simulink model "KUKA_EE_Trajectory_follower"  (R2021b)
settings: Solver=ode4  StartTime=0.0  StopTime=100  FixedStep=0.01  RelTol=1e-3
InitFcn:
  | %rho_0t=[0.29;0.29;0.29]; %m
  | %V_0t=[-0.001;-0.001;0];%[-0.0005;-0.0005;0];
  | %w_t=[0;0;-0.002];
  | 
  | 
  | %rho_0t=[0.3;0.3;0.2]; %m
  | %V_0t=[-0.001;-0.001;0];%[-0.0005;-0.0005;0];
  | %w_t=[0;0;-0.001];
values from neighbouring files (symbols this model uses):
  I0 = eye(3)*416.667    [Main.m]
  iota0 = eye(6,6)    [Internal_KUKA_Main.m]    (also in KUKA_Main.m; Main.m = [1 0 0; 0 1 0;zeros(3,3);0 0 1])
  K_d = 10*[1.3*eye(3) zeros(3);zeros(3) 0.8*eye(3)]    [Initiate_FQ.m]    (also in Internal_KUKA_Main.m = 200*[0.7*eye(3) zeros(3);zeros(3) 0.5*eye(3)]; KUKA_Main.m = [0.7*eye(3) zeros(3);zeros(3) 0.5*eye(3)])
  K_i = 5*[0.1*eye(3) zeros(3);zeros(3) 0.01*eye(3)]    [Initiate_FQ.m]    (also in Internal_KUKA_Main.m = 200*[0.01*eye(3) zeros(3);zeros(3) 0.001*eye(3)]; KUKA_Main.m = [0.01*eye(3) zeros(3);zeros(3) 0.001*eye(3)])
  K_p = 50*[0.1 0 0 0 0 0;0 0.1 0 0 0 0; 0 0 0.1 0 0 0; 0 0 0 0.01 0 0 ... (first row only)    [Initiate_FQ.m]    (also in Internal_KUKA_Main.m = 200*[0.1 0 0 0 0 0;0 0.1 0 0 0 0; 0 0 0.1 0 0 0; 0 0 0 0.01 ; KUKA_Main.m = [0.1 0 0 0 0 0;0 0.1 0 0 0 0; 0 0 0.1 0 0 0; 0 0 0 0.01 0 0)
  K_w = 20*eye(7)    [Initiate_FQ.m]
  K_wd = 1*eye(7)    [Initiate_FQ.m]
  M0 = M_temp.M0.data(:,:,1)    [Initiate_FQ.m]    (also in Internal_KUKA_Main.m; KUKA_Main.m)
  m0 = robot.Bodies{1,n+1}.Mass    [Internal_KUKA_Main.m]    (also in KUKA_Main.m; Main.m = 100)
  M0m = M_temp.M0m.data(:,:,1)    [Initiate_FQ.m]    (also in Internal_KUKA_Main.m; KUKA_Main.m)
  M_t = [eye(3)*mt zeros(3); zeros(3) eye(3)*0.416667]    [Initiate_FQ.m]    (also in Internal_KUKA_Main.m = [eye(3)*mt zeros(3); zeros(3) eye(3)*80]; KUKA_Main.m = [eye(3)*mt zeros(3); zeros(3) eye(3)*80])
  Mm = simplify(transpose(Xi_m)*transpose(Lm)*diagM*Lm*Xi_m)    [Internal_KUKA_Main.m]    (also in KUKA_Main.m)
  mm = zeros(1,n)    [Internal_KUKA_Main.m]    (also in KUKA_Main.m; Main.m = [2 2])
  mu = -10.*P0    [Initiate_FQ.m]    (also in Internal_KUKA_Main.m = P; KUKA_Main.m = P; Main.m = zeros(6,1)')
  mu_t = -10.*M_t*[V_0t;w_t]    [Initiate_FQ.m]    (also in Internal_KUKA_Main.m = M_t*[V_0t;w_t]; KUKA_Main.m = M_t*[V_0t;w_t])
  q_dot_m = 0.01*q_dot_m    [Initiate_FQ.m]    (also in Internal_KUKA_Main.m = [qdot1;qdot2;qdot3;qdot4;qdot5;qdot6;qdot7]; KUKA_Main.m = [qdot1;qdot2;qdot3;qdot4;qdot5;qdot6;qdot7]; Main.m = [0;0]; sendJointTorques.m = fread(t, 7, 'double'))
  q_m = [0.2;1.2;0.3;1.8;0.5;1.3;0.6]    [Initiate_FQ.m]    (also in Internal_KUKA_Main.m = [q_m1;q_m2;q_m3;q_m4;q_m5;q_m6;q_m7]; KUKA_Main.m = [q_m1;q_m2;q_m3;q_m4;q_m5;q_m6;q_m7]; Main.m = [0;0]; sendJointTorques.m = fread(t, 7, 'double'))
  rho_0t = [0;0;0.2]    [Initiate_FQ.m]    (also in Internal_KUKA_Main.m = [0.24;0.26;0.25]; KUKA_Main.m = [0.23;0.27;0.26])
  sc_size = 0    [Internal_KUKA_Main.m]    (also in KUKA_Main.m = 1)
  V_0t = -[-0.0005;-0.0005;0]    [Initiate_FQ.m]    (also in Internal_KUKA_Main.m = [-0.01;-0.01;0]; KUKA_Main.m = [-0.002;-0.002;0])
  V_I0 = 0.01*V_I0    [Initiate_FQ.m]    (also in Internal_KUKA_Main.m = [0;0;0;0;0;0]; KUKA_Main.m = [0;0;0;0;0;0]; Main.m = [0;0;0])
  X = [0 -x(3) x(2) ; x(3) 0 -x(1) ; -x(2) x(1) 0 ]    [skewsym.m]
  Xi_m = Xi_m(1:robot.n*6,1:robot.n)    [Internal_KUKA_Main.m]    (also in KUKA_Main.m)
  Xi_m_matrix = zeros(6*n,n)    [Internal_KUKA_Main.m]    (also in KUKA_Main.m; Main.m)
undefined symbols (not defined in the file or in its folder): fall_distance, g_cm, g_cm0, Ie, Im, m0_frak, m_diag, me, rise_time, Y, Z
libraries: nesl_utility x178, sm_lib x175, robotcorelib x7
(part 4 of 8)

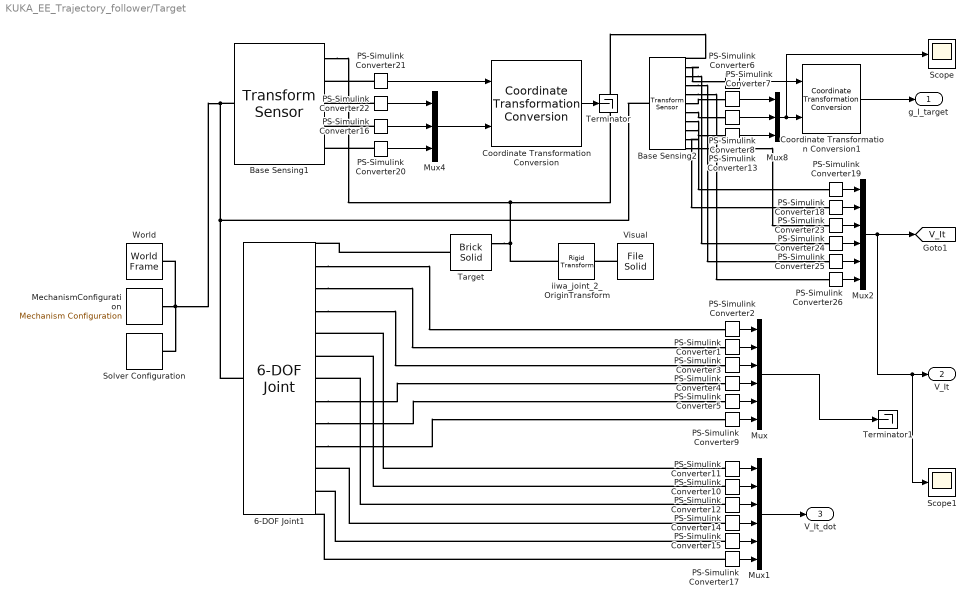
== system KUKA_EE_Trajectory_follower/Target ==
  6-DOF Joint1 : sm_lib/Joints/6-DOF Joint  JointMode=Normal  SenseConstraintForce=off  SenseConstraintForceX=off  SenseConstraintForceY=off  SenseConstraintForceZ=off  SenseConstraintTorque=off  SenseConstraintTorqueX=off  SenseConstraintTorqueY=off  SenseConstraintTorqueZ=off  SenseTotalForce=off  SenseTotalForceX=off  SenseTotalForceY=off  SenseTotalForceZ=off  SenseTotalTorque=off  SenseTotalTorqueX=off  SenseTotalTorqueY=off  SenseTotalTorqueZ=off  CompositeWrenchDir=FollowerOnBase  CompositeWrenchFrame=BaseFrame  PxEquilibriumPosition=0  PxEquilibriumPositionUnits=m  PxSpringStiffness=0  PxSpringStiffnessUnits=N/m  PxDampingCoefficient=0  PxDampingCoefficientUnits=N/(m/s)  PxTorqueActuationMode=NoTorque  PxMotionActuationMode=ComputedMotion  PxSensePosition=off  PxSenseVelocity=on  PxSenseAcceleration=on  PxSenseTorqueForce=off  PxSenseLowerLimitTorqueForce=off  PxSenseUpperLimitTorqueForce=off  PxLowerLimitSpecify=off  PxLowerLimitBound=-1  PxLowerLimitBoundUnits=m  PxLowerLimitStiffness=1e6  PxLowerLimitStiffnessUnits=N/m  PxLowerLimitDamping=1e3  PxLowerLimitDampingUnits=N/(m/s)  PxLowerLimitTransitionRegionWidth=1e-4  PxLowerLimitTransitionRegionWidthUnits=m  PxUpperLimitSpecify=off  PxUpperLimitBound=1  PxUpperLimitBoundUnits=m  PxUpperLimitStiffness=1e6  PxUpperLimitStiffnessUnits=N/m  PxUpperLimitDamping=1e3  PxUpperLimitDampingUnits=N/(m/s)  PxUpperLimitTransitionRegionWidth=1e-4  PxUpperLimitTransitionRegionWidthUnits=m  PxPositionTargetSpecify=on  PxPositionTargetPriority=High  PxPositionTargetValue=rho_0t(1)  PxPositionTargetValueUnits=m  PxVelocityTargetSpecify=on  PxVelocityTargetPriority=High  PxVelocityTargetValue=V_0t(1)  PxVelocityTargetValueUnits=m/s  PyEquilibriumPosition=0  PyEquilibriumPositionUnits=m  PySpringStiffness=0  PySpringStiffnessUnits=N/m  PyDampingCoefficient=0  PyDampingCoefficientUnits=N/(m/s)  PyTorqueActuationMode=NoTorque  PyMotionActuationMode=ComputedMotion  PySensePosition=off  PySenseVelocity=on  PySenseAcceleration=on  PySenseTorqueForce=off  PySenseLowerLimitTorqueForce=off  PySenseUpperLimitTorqueForce=off  PyLowerLimitSpecify=off  PyLowerLimitBound=-1  PyLowerLimitBoundUnits=m  PyLowerLimitStiffness=1e6  PyLowerLimitStiffnessUnits=N/m  PyLowerLimitDamping=1e3  PyLowerLimitDampingUnits=N/(m/s)  PyLowerLimitTransitionRegionWidth=1e-4  PyLowerLimitTransitionRegionWidthUnits=m  PyUpperLimitSpecify=off  PyUpperLimitBound=1  PyUpperLimitBoundUnits=m  PyUpperLimitStiffness=1e6  PyUpperLimitStiffnessUnits=N/m  PyUpperLimitDamping=1e3  PyUpperLimitDampingUnits=N/(m/s)  PyUpperLimitTransitionRegionWidth=1e-4  PyUpperLimitTransitionRegionWidthUnits=m  PyPositionTargetSpecify=on  PyPositionTargetPriority=High  PyPositionTargetValue=rho_0t(2)  PyPositionTargetValueUnits=m  PyVelocityTargetSpecify=on  PyVelocityTargetPriority=High  PyVelocityTargetValue=V_0t(2)  PyVelocityTargetValueUnits=m/s  PzEquilibriumPosition=0  PzEquilibriumPositionUnits=m  PzSpringStiffness=0  PzSpringStiffnessUnits=N/m  PzDampingCoefficient=0  PzDampingCoefficientUnits=N/(m/s)  PzTorqueActuationMode=NoTorque  PzMotionActuationMode=ComputedMotion  PzSensePosition=off  PzSenseVelocity=on  PzSenseAcceleration=on  PzSenseTorqueForce=off  PzSenseLowerLimitTorqueForce=off  PzSenseUpperLimitTorqueForce=off  PzLowerLimitSpecify=off  PzLowerLimitBound=-1  PzLowerLimitBoundUnits=m  PzLowerLimitStiffness=1e6  PzLowerLimitStiffnessUnits=N/m  PzLowerLimitDamping=1e3  PzLowerLimitDampingUnits=N/(m/s)  PzLowerLimitTransitionRegionWidth=1e-4  PzLowerLimitTransitionRegionWidthUnits=m  PzUpperLimitSpecify=off  PzUpperLimitBound=1  PzUpperLimitBoundUnits=m  PzUpperLimitStiffness=1e6  PzUpperLimitStiffnessUnits=N/m  PzUpperLimitDamping=1e3  PzUpperLimitDampingUnits=N/(m/s)  PzUpperLimitTransitionRegionWidth=1e-4  PzUpperLimitTransitionRegionWidthUnits=m  PzPositionTargetSpecify=on  PzPositionTargetPriority=High  PzPositionTargetValue=rho_0t(3)  PzPositionTargetValueUnits=m  PzVelocityTargetSpecify=on  PzVelocityTargetPriority=High  PzVelocityTargetValue=V_0t(3)  PzVelocityTargetValueUnits=m/s  SphDefPosRotationMethod=None  SphDefPosRotationAngleUnits=deg  SphDefPosRotationStandardAxis=+Z  SphDefPosRotationAngle=0.0  SphDefPosRotationArbitraryAxis=[0 0 1]  SphDefPosFollAlignAxisA=+X  SphDefPosBaseAlignAxisA=+Y  SphDefPosFollAlignAxisB=+Y  SphDefPosBaseAlignAxisB=+Z  SphDefPosRotationSequenceAxes=FollowerAxes  SphDefPosRotationSequence=XYX  SphDefPosRotationSequenceAngles=[0 0 0]  SphDefPosRotationSequenceAnglesUnits=deg  SphDefPosRotationMatrix=[1 0 0; 0 1 0; 0 0 1]  SphEqPosRotationMethod=None  SphEqPosRotationAngleUnits=deg  SphEqPosRotationStandardAxis=+Z  SphEqPosRotationAngle=0.0  SphEqPosRotationArbitraryAxis=[0 0 1]  SphEqPosFollAlignAxisA=+X  SphEqPosBaseAlignAxisA=+Y  SphEqPosFollAlignAxisB=+Y  SphEqPosBaseAlignAxisB=+Z  SphEqPosRotationSequenceAxes=FollowerAxes  SphEqPosRotationSequence=XYX  SphEqPosRotationSequenceAngles=[0 0 0]  SphEqPosRotationSequenceAnglesUnits=deg  SphEqPosRotationMatrix=[1 0 0; 0 1 0; 0 0 1]  SphSpringStiffness=0  SphSpringStiffnessUnits=N*m/deg  SphDampingCoefficient=0  SphDampingCoefficientUnits=N*m/(deg/s)  SphActuateTorqueX=off  SphActuateTorqueY=off  SphActuateTorqueZ=off  SphActuateTorque=off  SphTorqueActuationMode=NoTorque  SphMotionActuationMode=ComputedMotion  SphActuationFrame=BaseFrame  SphSensePosition=off  SphSenseVelocityX=on  SphSenseVelocityY=on  SphSenseVelocityZ=on  SphSenseVelocity=off  SphSenseAccelerationX=on  SphSenseAccelerationY=on  SphSenseAccelerationZ=on  SphSenseAcceleration=off  SphSenseTorqueX=off  SphSenseTorqueY=off  SphSenseTorqueZ=off  SphSenseTorqueForce=off  SphSenseLowerLimitTorqueMag=off  SphSenseUpperLimitTorqueMag=off  SphSensingFrame=BaseFrame  SphLowerLimitSpecify=off  SphLowerLimitBound=15  SphLowerLimitBoundUnits=deg  SphLowerLimitStiffness=1e4  SphLowerLimitStiffnessUnits=N*m/deg  SphLowerLimitDamping=10  SphLowerLimitDampingUnits=N*m/(deg/s)  SphLowerLimitTransitionRegionWidth=0.1  SphLowerLimitTransitionRegionWidthUnits=deg  SphUpperLimitSpecify=off  SphUpperLimitBound=45  SphUpperLimitBoundUnits=deg  SphUpperLimitStiffness=1e4  SphUpperLimitStiffnessUnits=N*m/deg  SphUpperLimitDamping=10  SphUpperLimitDampingUnits=N*m/(deg/s)  SphUpperLimitTransitionRegionWidth=0.1  SphUpperLimitTransitionRegionWidthUnits=deg  SphPositionTargetRotationMethod=RotationSequence  SphPositionTargetRotationAngleUnits=deg  SphPositionTargetRotationStandardAxis=+Z  SphPositionTargetRotationAngle=0.0  SphPositionTargetRotationArbitraryAxis=[0 0 1]  SphPositionTargetFollAlignAxisA=+X  SphPositionTargetBaseAlignAxisA=+Y  SphPositionTargetFollAlignAxisB=+Y  SphPositionTargetBaseAlignAxisB=+Z  SphPositionTargetRotationSequenceAxes=FollowerAxes  SphPositionTargetRotationSequence=XYZ  SphPositionTargetRotationSequenceAngles=[0 0 0]  SphPositionTargetRotationSequenceAnglesUnits=deg  SphPositionTargetRotationMatrix=[1 0 0; 0 1 0; 0 0 1]  SphPositionTargetSpecify=on  SphPositionTargetPriority=High  SphVelocityTargetValue=w_t  SphVelocityTargetValueUnits=rad/s  SphVelocityTargetSpecify=on  SphVelocityTargetPriority=High  SphVelocityTargetInFollowerFrame=off
  Base Sensing1 : sm_lib/Frames and Transforms/Transform Sensor  MeasurementFrame=Base  SenseAngle=off  SenseAxis=off  SenseAngle1=off  SenseAngle2=off  SenseAngle3=off  SenseQ=off  SenseR=on  SenseOmegaX=off  SenseOmegaY=off  SenseOmegaZ=off  SenseOmega1=off  SenseOmega2=off  SenseOmega3=off  SenseQDot=off  SenseRDot=off  SenseAlphaX=off  SenseAlphaY=off  SenseAlphaZ=off  SenseAlpha1=off  SenseAlpha2=off  SenseAlpha3=off  SenseQDDot=off  SenseRDDot=off  SenseX=on  SenseY=on  SenseZ=on  SenseRad=off  SenseAzim=off  SenseDist=off  SenseInc=off  SenseXDot=off  SenseYDot=off  SenseZDot=off  SenseRadDot=off  SenseAzimDot=off  SenseDistDot=off  SenseIncDot=off  SenseXDDot=off  SenseYDDot=off  SenseZDDot=off  SenseRadDDot=off  SenseAzimDDot=off  SenseDistDDot=off  SenseIncDDot=off
  Base Sensing2 : sm_lib/Frames and Transforms/Transform Sensor  MeasurementFrame=Base  SenseAngle=off  SenseAxis=off  SenseAngle1=off  SenseAngle2=off  SenseAngle3=off  SenseQ=off  SenseR=on  SenseOmegaX=on  SenseOmegaY=on  SenseOmegaZ=on  SenseOmega1=off  SenseOmega2=off  SenseOmega3=off  SenseQDot=off  SenseRDot=off  SenseAlphaX=off  SenseAlphaY=off  SenseAlphaZ=off  SenseAlpha1=off  SenseAlpha2=off  SenseAlpha3=off  SenseQDDot=off  SenseRDDot=off  SenseX=on  SenseY=on  SenseZ=on  SenseRad=off  SenseAzim=off  SenseDist=off  SenseInc=off  SenseXDot=on  SenseYDot=on  SenseZDot=on  SenseRadDot=off  SenseAzimDot=off  SenseDistDot=off  SenseIncDot=off  SenseXDDot=off  SenseYDDot=off  SenseZDDot=off  SenseRadDDot=off  SenseAzimDDot=off  SenseDistDDot=off  SenseIncDDot=off
  Coordinate Transformation Conversion : robotcorelib/Coordinate Transformation Conversion  InputRepresentation=Rotation Matrix  InputEulerSequence=ZYX  ShowTrVecInputPort=on  OutputRepresentation=Homogeneous Transformation  OutputEulerSequence=ZYX  ShowTrVecOutputPort=on  SimulateUsing=Interpreted execution
      settings: SourceProductBaseCode=NV,RO,RR,UV
  Coordinate Transformation Conversion1 : robotcorelib/Coordinate Transformation Conversion  InputRepresentation=Rotation Matrix  InputEulerSequence=ZYX  ShowTrVecInputPort=on  OutputRepresentation=Homogeneous Transformation  OutputEulerSequence=ZYX  ShowTrVecOutputPort=on  SimulateUsing=Interpreted execution
      settings: SourceProductBaseCode=NV,RO,RR,UV
  MechanismConfiguration : sm_lib/Utilities/Mechanism Configuration  UniformGravity=Constant  GravityVector=[0 0 0]  GravityUnits=m/s^2  LinearizationDelta=0.001  JointModeTransitionNonlinearIterations=2
  Mux : Mux  Inputs=6
  Mux1 : Mux  Inputs=6
  Mux2 : Mux  Inputs=6
  Mux4 : Mux  Inputs=3
  Mux8 : Mux  Inputs=3
  PS-Simulink Converter{1..26} (26 alike) : nesl_utility/PS-Simulink Converter  PhysicalDomain=network_engine_domain  SubClassName=ps_output  LeftPortType=input  RightPortType=output  PseudoPeriodic=off  Frequencies=[]  Unit=inherit  AffineConversion=off
      settings: SourceProductBaseCode=PW,SS
  Scope : Scope
  Scope1 : Scope
  Solver Configuration : nesl_utility/Solver Configuration  PhysicalDomain=network_engine_domain  SubClassName=solver  LeftPortType=input  RightPortType=generic  Tones=[]  Harmonics=[]  SimulateNoise=off  Profile=off  UseLocalSampling=off  EnableSwitchedLinearOptims=on  FrequencyDomain=off  UseCCode=off  RelTol=0.001  AbsTol=0.001  MinStep=1e-09  ToWorkspace=off  RevertToSquareIcSolve=off  NumHomotopyIterations=100  PhasorMode=off  PhasorModeNumHarmonics=1  DoDC=off  ResidualTolerance=1e-09  UseLocalSolver=off  LocalSolverChoice=NE_BACKWARD_EULER_ADVANCER  LocalSolverSampleTime=0.001  DoFixedCost=off  MaxNonlinIter=3  MaxModeIter=2  ComputeImpulses=off  ImpulseIterations=2  LinearAlgebra=Full  EquationFormulation=NE_TIME_EF  DelaysMemoryBudget=1024  AutomaticFiltering=on  FilteringTimeConstant=0.001  PartitionStorageMethod=AS_NEEDED  PartitionMemoryBudget=1024  PartitionMethod=ROBUST
      settings: SourceProductBaseCode=PW,SS
  Target : sm_lib/Body Elements/Brick Solid  GraphicAmbientColor=[0.15 0.15 0.15 1.0]  BasedOnType=Mass  BrickDimensions=[0.5, 0.5, 0.5]  BrickDimensionUnits=m  CenterOfMass=[0 0 0]  CenterOfMassUnits=m  GraphicDiffuseColor=[0.5 0.5 0.5]  Density=1000  DensityUnits=kg/m^3  DoExposeReferenceFrame=on  GraphicEmissiveColor=[0.0 0.0 0.0 1.0]  ExportEntireGeometry=on  SerializedFrames=<Frames><Frame><Id>Frame1</Id><Value><Name>F1</Name><Origin><Source>GeometricFeature</Source><FeatureName>-x -y -z point</FeatureName></Origin><PrimaryAxis><DefinedDirection>+Z</DefinedDirection><Source>ReferenceFrame</Source><SourceDirection>+Z</SourceDirection><FeatureName></FeatureName></PrimaryAxis><SecondaryAxis><DefinedDirection>+X</DefinedDirection><Source>ReferenceFrame</Source><SourceDirection>+X</SourceDirection><FeatureName></FeatureName></SecondaryAxis></Value></Frame></Frames>  MarkerShape=Sphere  MarkerSize=10  GraphicType=None  InertiaType=CalculateFromGeometry  Mass=10  MassUnits=kg  MomentsOfInertia=[1 1 1]  MomentsOfInertiaUnits=kg*m^2  GraphicOpacity=1.0  ProductsOfInertia=[0 0 0]  ProductsOfInertiaUnits=kg*m^2  GraphicShininess=75  GraphicSpecularColor=[0.5 0.5 0.5 1.0]  GraphicVisPropType=SimpleVisualProperties
  Terminator : Terminator
  Terminator1 : Terminator
  Visual : sm_lib/Body Elements/File Solid  ExtGeomFileName=Spacecrafts/CubeSatAssembly.stl  UnitType=Custom  ExtGeomFileUnits=cm  StepReaderType=HEX  ExportConvexHullGeometry=off  InertiaType=Custom  Mass=0  MassUnits=kg  CenterOfMass=[0, 0, 0]  CenterOfMassUnits=m  MomentsOfInertia=[0, 0, 0]  MomentsOfInertiaUnits=kg*m^2  ProductsOfInertia=[0, 0, 0]  ProductsOfInertiaUnits=kg*m^2  BasedOnType=DensityFromFile  Density=1000  DensityUnits=kg/m^3  DoExposeReferenceFrame=on  SerializedFrames=<Frames/>  GraphicType=FromGeometry  MarkerShape=Sphere  MarkerSize=10  GraphicVisPropType=SimpleVisualProperties  GraphicDiffuseColor=[0.4 0.4 0.4]  GraphicSpecularColor=[0.5 0.5 0.5 1.0]  GraphicAmbientColor=[0.15 0.15 0.15 1.0]  GraphicEmissiveColor=[0.0 0.0 0.0 1.0]  GraphicShininess=75  GraphicOpacity=1
  World : sm_lib/Frames and Transforms/World Frame
  iiwa_joint_2_OriginTransform : sm_lib/Frames and Transforms/Rigid Transform  TranslationMethod=Cartesian  TranslationStandardOffset=0  TranslationLengthUnit=m  TranslationStandardAxis=+Z  TranslationCartesianOffset=[-3.28, -4.43, 0.817]  TranslationROffset=0  TranslationROffsetUnits=m  TranslationZOffset=0  TranslationZOffsetUnits=m  TranslationThetaOffset=0  TranslationThetaOffsetUnits=deg  RotationMethod=RotationSequence  RotationAngleUnits=deg  RotationStandardAxis=+Z  RotationAngle=0.0  RotationArbitraryAxis=[0 0 1]  FollAlignAxisA=+X  BaseAlignAxisA=+Y  FollAlignAxisB=+Y  BaseAlignAxisB=+Z  RotationSequenceAxes=FollowerAxes  RotationSequence=XYZ  RotationSequenceAngles=[0 0 0]  RotationSequenceAnglesUnits=rad  RotationMatrix=[1 0 0; 0 1 0; 0 0 1]
  g_I_target : Outport
  V_It : Outport  Port=2
  V_It_dot : Outport  Port=3
  tag scope: V_It=global
  wires:
  PS-Simulink Converter20/1 -> Mux4/3
  PS-Simulink Converter13/1 -> Mux8/3
  PS-Simulink Converter4/1 -> Mux/4
  PS-Simulink Converter9/1 -> Mux/6
  PS-Simulink Converter3/1 -> Mux/3
  Coordinate Transformation Conversion/1 -> Terminator/1
  Mux1/1 -> V_It_dot/1
  PS-Simulink Converter16/1 -> Mux4/2
  Coordinate Transformation Conversion1/1 -> g_I_target/1
  PS-Simulink Converter11/1 -> Mux1/1
  PS-Simulink Converter1/1 -> Mux/2
  PS-Simulink Converter15/1 -> Mux1/5
  PS-Simulink Converter14/1 -> Mux1/4
  PS-Simulink Converter2/1 -> Mux/1
  PS-Simulink Converter7/1 -> Mux8/1
  PS-Simulink Converter21/1 -> Coordinate Transformation Conversion/1
  PS-Simulink Converter10/1 -> Mux1/2
  PS-Simulink Converter6/1 -> Coordinate Transformation Conversion1/1
  PS-Simulink Converter17/1 -> Mux1/6
  Mux4/1 -> Coordinate Transformation Conversion/2
  PS-Simulink Converter12/1 -> Mux1/3
  PS-Simulink Converter5/1 -> Mux/5
  PS-Simulink Converter22/1 -> Mux4/1
  PS-Simulink Converter8/1 -> Mux8/2
  Mux8/1 -> Scope/1, Coordinate Transformation Conversion1/2
  PS-Simulink Converter24/1 -> Mux2/4
  PS-Simulink Converter18/1 -> Mux2/2
  PS-Simulink Converter25/1 -> Mux2/5
  Mux2/1 -> Scope1/1, V_It/1, [V_It]
  PS-Simulink Converter19/1 -> Mux2/1
  PS-Simulink Converter23/1 -> Mux2/3
  PS-Simulink Converter26/1 -> Mux2/6
  Mux/1 -> Terminator1/1
  connections:
  Target/RConn1 -- 6-DOF Joint1/RConn1
  Base Sensing2/RConn2 -- PS-Simulink Converter6/LConn1
  PS-Simulink Converter15/LConn1 -- 6-DOF Joint1/RConn12
  6-DOF Joint1/RConn10 -- PS-Simulink Converter9/LConn1
  PS-Simulink Converter10/LConn1 -- 6-DOF Joint1/RConn6
  PS-Simulink Converter22/LConn1 -- Base Sensing1/RConn3
  Base Sensing2/RConn3 -- PS-Simulink Converter24/LConn1
  PS-Simulink Converter20/LConn1 -- Base Sensing1/RConn5
  World/RConn1 -- Base Sensing2/LConn1 -- 6-DOF Joint1/LConn1 -- Base Sensing1/LConn1 -- MechanismConfiguration/RConn1 -- Solver Configuration/RConn1
  PS-Simulink Converter21/LConn1 -- Base Sensing1/RConn2
  PS-Simulink Converter16/LConn1 -- Base Sensing1/RConn4
  Base Sensing2/RConn5 -- PS-Simulink Converter26/LConn1
  PS-Simulink Converter12/LConn1 -- 6-DOF Joint1/RConn7
  6-DOF Joint1/RConn9 -- PS-Simulink Converter5/LConn1
  6-DOF Joint1/RConn2 -- PS-Simulink Converter2/LConn1
  PS-Simulink Converter17/LConn1 -- 6-DOF Joint1/RConn13
  6-DOF Joint1/RConn4 -- PS-Simulink Converter3/LConn1
  PS-Simulink Converter14/LConn1 -- 6-DOF Joint1/RConn11
  6-DOF Joint1/RConn8 -- PS-Simulink Converter4/LConn1
  PS-Simulink Converter11/LConn1 -- 6-DOF Joint1/RConn5
  6-DOF Joint1/RConn3 -- PS-Simulink Converter1/LConn1
  Visual/RConn1 -- iiwa_joint_2_OriginTransform/RConn1
  Base Sensing2/RConn4 -- PS-Simulink Converter25/LConn1
  Base Sensing2/RConn6 -- PS-Simulink Converter7/LConn1
  Base Sensing2/RConn7 -- PS-Simulink Converter8/LConn1
  Base Sensing2/RConn8 -- PS-Simulink Converter13/LConn1
  Base Sensing2/RConn9 -- PS-Simulink Converter19/LConn1
  Base Sensing2/RConn10 -- PS-Simulink Converter18/LConn1
  Base Sensing2/RConn11 -- PS-Simulink Converter23/LConn1
  iiwa_joint_2_OriginTransform/LConn1 -- Target/LConn1 -- Base Sensing1/RConn1 -- Base Sensing2/RConn1

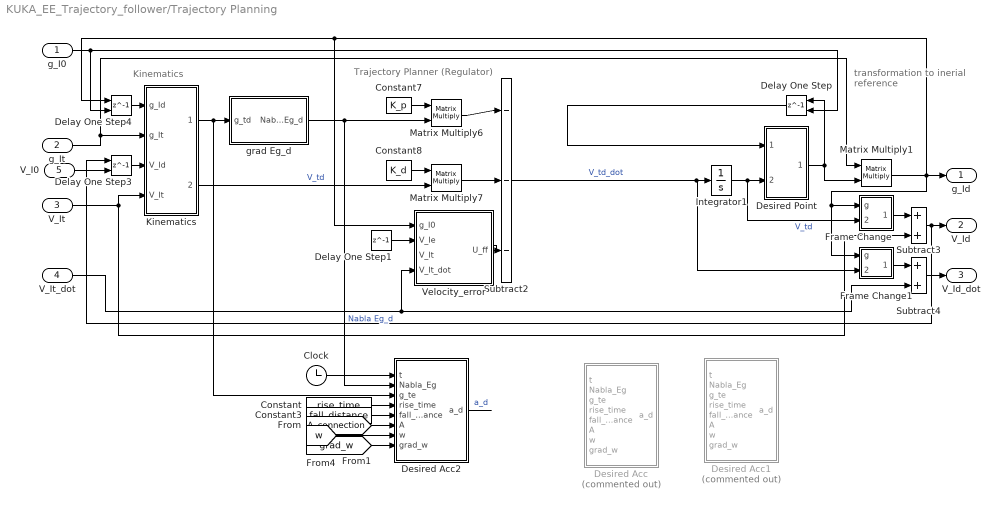
== system KUKA_EE_Trajectory_follower/Trajectory Planning ==
  note: Trajectory Planner (Regulator)
  note: Kinematics
  note: transformation
      | to inerial reference
  g_I0 : Inport
  g_It : Inport  Port=2
  V_It : Inport  Port=3
  V_It_dot : Inport  Port=4
  V_I0 : Inport  Port=5
  Clock : Clock
  Constant : Constant  Value=rise_time
  Constant3 : Constant  Value=fall_distance
  Constant7 : Constant  Value=K_p
  Constant8 : Constant  Value=K_d
  Delay One Step{,1,3..4} (4 alike) : Delay  DelayLength=1  InitialConditionSource=Input port
      settings: InputPortMap=u0,p4
  Desired Acc : MATLAB Function  Commented=on  TreatAsAtomicUnit=on
  Desired Acc1 : MATLAB Function  Commented=on  TreatAsAtomicUnit=on
  Desired Acc2 : MATLAB Function  TreatAsAtomicUnit=on
  Desired Point : MATLAB Function  TreatAsAtomicUnit=on
  Frame Change : MATLAB Function  TreatAsAtomicUnit=on
  Frame Change1 : MATLAB Function  TreatAsAtomicUnit=on
  Integrator1 : Integrator
  Kinematics : Subsystem
  Matrix Multiply1 : Product  Multiplication=Matrix(*)
  Matrix Multiply6 : Product  Multiplication=Matrix(*)
  Matrix Multiply7 : Product  Multiplication=Matrix(*)
  Subtract2 : Sum  Inputs=---
  Subtract3 : Sum
  Subtract4 : Sum
  Velocity_error : MATLAB Function  TreatAsAtomicUnit=on
  grad Eg_d : MATLAB Function  TreatAsAtomicUnit=on
  g_Id : Outport
  V_Id : Outport  Port=2
  V_Id_dot : Outport  Port=3
  wires:
  Constant3/1 -> Desired Acc2/5(fall_distance)
  Clock/1 -> Desired Acc2/1(t)
  [A_connection] -> Desired Acc2/6(A)
  [grad_w] -> Desired Acc2/8(grad_w)
  Constant/1 -> Desired Acc2/4(rise_time)
  Desired Acc2/1(a_d) -> ?  "a_d"
  [w] -> Desired Acc2/7(w)
  Kinematics/1(g_td) -> Desired Acc2/3(g_te), grad Eg_d/1(g_td)
  V_It/1 -> Subtract3/2, Kinematics/4(V_It)
  grad Eg_d/1(Nabla_Eg_d) -> Desired Acc2/2(Nabla_Eg), Matrix Multiply6/2  "Nabla Eg_d"
  g_It/1 -> Matrix Multiply1/1, Kinematics/2(g_It)
  Delay One Step3/1 -> Kinematics/3(V_Id)
  Kinematics/2(V_td) -> Matrix Multiply7/2  "V_td"
  Delay One Step/1 -> Desired Point/1(g_prev)
  V_I0/1 -> Delay One Step3/2
  Velocity_error/1(U_ff) -> Subtract2/3
  Constant8/1 -> Matrix Multiply7/1
  Matrix Multiply7/1 -> Subtract2/2
  Constant7/1 -> Matrix Multiply6/1
  V_It_dot/1 -> Velocity_error/4(V_It_dot), Subtract4/2
  Integrator1/1 -> Desired Point/2(V_d), Frame Change/2(A_in)  "V_td"
  g_I0/1 -> Delay One Step4/2, Delay One Step/2
  Matrix Multiply6/1 -> Subtract2/1
  Subtract2/1 -> Frame Change1/2(A_in), Integrator1/1  "V_td_dot"
  Desired Point/1(g_td) -> Matrix Multiply1/2, Delay One Step/1
  Delay One Step1/1 -> Velocity_error/2(V_Ie)
  Subtract3/1 -> Delay One Step3/1, V_Id/1
  Subtract4/1 -> V_Id_dot/1
  Matrix Multiply1/1 -> Velocity_error/1(g_I0), Delay One Step4/1, Frame Change1/1(g), Frame Change/1(g), g_Id/1
  Delay One Step4/1 -> Kinematics/1(g_Id)
  Frame Change/1(A_out) -> Subtract3/1
  Frame Change1/1(A_out) -> Subtract4/1

== system KUKA_EE_Trajectory_follower/Dynamic Parameters/A_connection1 ==
  M0 : Inport
  M0m : Inport  Port=2
  Divide : Product  Inputs=/*  Multiplication=Matrix(*)
  A : Outport
  wires:
  Divide/1 -> A/1
  M0/1 -> Divide/1
  M0m/1 -> Divide/2

== system KUKA_EE_Trajectory_follower/Dynamic Parameters/Mass Matrix Blocks1 ==
  Lm : Inport
  Lm0 : Inport  Port=2
  Xi_m_matrix : Inport  Port=3
  Add : Sum
  Constant1 : Constant  Value=m0_frak  VectorParams1D=off
  Constant2 : Constant  Value=m_diag  VectorParams1D=off
  Matrix Multiply1 : Product  Inputs=4  Multiplication=Matrix(*)
  Matrix Multiply3 : Product  Inputs=5  Multiplication=Matrix(*)
  Matrix Multiply4 : Product  Inputs=3  Multiplication=Matrix(*)
  Matrix Multiply5 : Product  Inputs=1  Multiplication=Matrix(*)
  Transpose3 : Math  Operator=transpose  SaturateOnIntegerOverflow=on
  Transpose4 : Math  Operator=transpose  SaturateOnIntegerOverflow=on
  Transpose5 : Math  Operator=transpose  SaturateOnIntegerOverflow=on
  M0 : Outport
  M0m : Outport  Port=2
  Mm : Outport  Port=3
  tag scope: diag_Mm=global
  wires:
  Xi_m_matrix/1 -> Matrix Multiply1/4, Matrix Multiply3/5, Transpose3/1
  Matrix Multiply5/1 -> M0/1
  Lm0/1 -> Transpose5/1, Matrix Multiply4/3
  Transpose5/1 -> Matrix Multiply4/1, Matrix Multiply1/1
  Transpose4/1 -> Matrix Multiply3/2
  Matrix Multiply3/1 -> Mm/1
  Matrix Multiply1/1 -> M0m/1
  Matrix Multiply4/1 -> Add/2
  Transpose3/1 -> Matrix Multiply3/1
  Lm/1 -> Matrix Multiply1/3, Matrix Multiply3/4, Transpose4/1
  Add/1 -> Matrix Multiply5/1
  Constant2/1 -> Matrix Multiply4/2, Matrix Multiply3/3, Matrix Multiply1/2, [diag_Mm]
  Constant1/1 -> Add/1

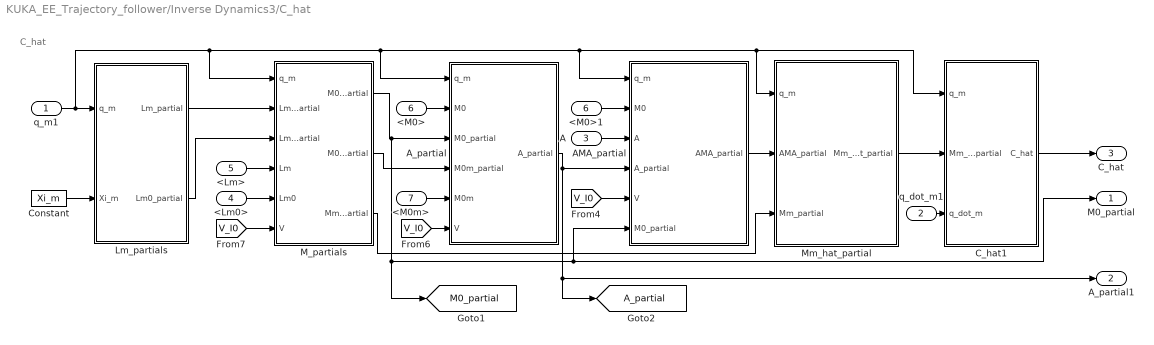
== system KUKA_EE_Trajectory_follower/Inverse Dynamics3/C_hat ==
  note: C_hat
  q_m1 : Inport
  q_dot_m1 : Inport  Port=2
  A : Inport  Port=3
  <Lm0> : Inport  Port=4
  <Lm> : Inport  Port=5
  <M0> : Inport  Port=6
  <M0m> : Inport  Port=7
  <M0>1 : InportShadow  Port=6
  AMA_partial : MATLAB Function  TreatAsAtomicUnit=on
  A_partial : MATLAB Function  TreatAsAtomicUnit=on
  C_hat1 : MATLAB Function  TreatAsAtomicUnit=on
  Constant : Constant  Value=Xi_m
  Lm_partials : Subsystem
  M_partials : Subsystem
  Mm_hat_partial : MATLAB Function  TreatAsAtomicUnit=on
  M0_partial : Outport
  A_partial1 : Outport  Port=2
  C_hat : Outport  Port=3
  tag scope: A_partial=global, M0_partial=global
  wires:
  M_partials/3(Mm_partial) -> Mm_hat_partial/3(Mm_partial)
  Lm_partials/2(Lm0_partial) -> M_partials/3(Lm0_partial)
  q_m1/1 -> Lm_partials/1(q_m), Mm_hat_partial/1(q_m), C_hat1/1(q_m), AMA_partial/1(q_m), A_partial/1(q_m), M_partials/1(q_m)
  <M0m>/1 -> A_partial/5(M0m)
  Lm_partials/1(Lm_partial) -> M_partials/2(Lm_partial)
  M_partials/1(M0_partial) -> A_partial/3(M0_partial), M0_partial/1, AMA_partial/6(M0_partial), [M0_partial]
  A_partial/1(A_partial) -> AMA_partial/4(A_partial), [A_partial], A_partial1/1
  Constant/1 -> Lm_partials/2(Xi_m)
  M_partials/2(M0m_partial) -> A_partial/4(M0m_partial)
  Mm_hat_partial/1(Mm_hat_partial) -> C_hat1/2(Mm_hat_partial)
  q_dot_m1/1 -> C_hat1/3(q_dot_m)
  AMA_partial/1(AMA_partial) -> Mm_hat_partial/2(AMA_partial)
  <M0>/1 -> A_partial/2(M0)
  [V_I0] -> A_partial/6(V)
  [V_I0] -> M_partials/6(V)
  <Lm>/1 -> M_partials/4(Lm)
  [V_I0] -> AMA_partial/5(V)
  A/1 -> AMA_partial/3(A)
  C_hat1/1(C_hat) -> C_hat/1
  <M0>1/1 -> AMA_partial/2(M0)
  <Lm0>/1 -> M_partials/5(Lm0)

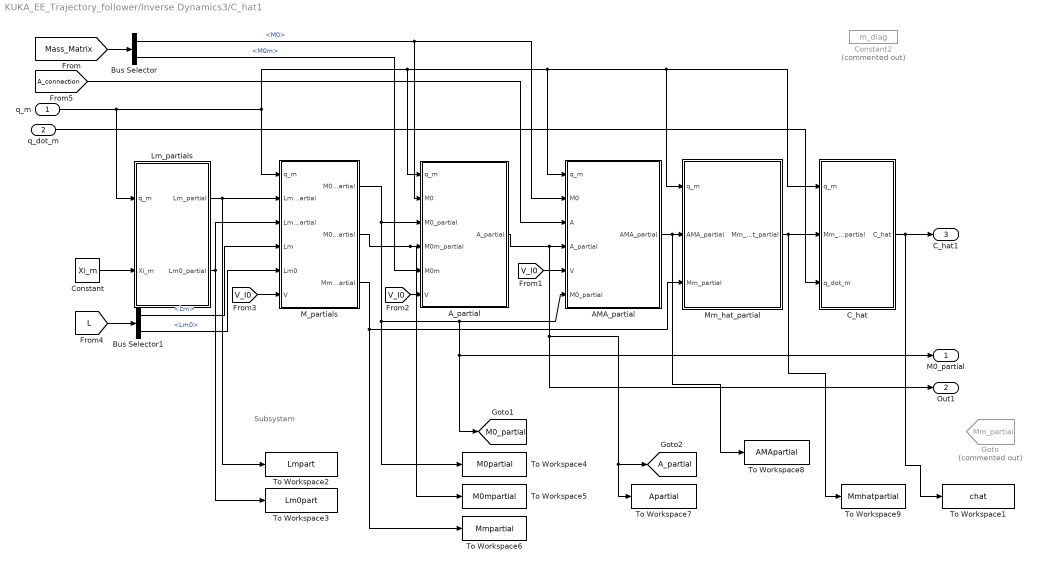
== system KUKA_EE_Trajectory_follower/Inverse Dynamics3/C_hat1 ==
  note: Subsystem
  q_m : Inport
  q_dot_m : Inport  Port=2
  AMA_partial : MATLAB Function  TreatAsAtomicUnit=on
  A_partial : MATLAB Function  TreatAsAtomicUnit=on
  Bus Selector : BusSelector  OutputSignals=M0,M0m
  Bus Selector1 : BusSelector  OutputSignals=Lm,Lm0
  C_hat : MATLAB Function  TreatAsAtomicUnit=on
  Constant : Constant  Value=Xi_m
  Constant2 : Constant  Commented=on  Value=m_diag  VectorParams1D=off
  Goto : Goto  Commented=on  GotoTag=Mm_partial  TagVisibility=global
  Lm_partials : Subsystem
  M_partials : Subsystem
  Mm_hat_partial : MATLAB Function  TreatAsAtomicUnit=on
  To Workspace1 : ToWorkspace  VariableName=chat  SaveFormat=Timeseries  SampleTime=-1
  To Workspace2 : ToWorkspace  VariableName=Lmpart  SaveFormat=Timeseries  SampleTime=-1
  To Workspace3 : ToWorkspace  VariableName=Lm0part  SaveFormat=Timeseries  SampleTime=-1
  To Workspace4 : ToWorkspace  VariableName=M0partial  SaveFormat=Timeseries  SampleTime=-1
  To Workspace5 : ToWorkspace  VariableName=M0mpartial  SaveFormat=Timeseries  SampleTime=-1
  To Workspace6 : ToWorkspace  VariableName=Mmpartial  SaveFormat=Timeseries  SampleTime=-1
  To Workspace7 : ToWorkspace  VariableName=Apartial  SaveFormat=Timeseries  SampleTime=-1
  To Workspace8 : ToWorkspace  VariableName=AMApartial  SaveFormat=Timeseries  SampleTime=-1
  To Workspace9 : ToWorkspace  VariableName=Mmhatpartial  SaveFormat=Timeseries  SampleTime=-1
  M0_partial : Outport
  Out1 : Outport  Port=2
  C_hat1 : Outport  Port=3
  tag scope: A_partial=global, M0_partial=global
  wires:
  [Mass_Matrix] -> Bus Selector/1
  Bus Selector/1 -> AMA_partial/2(M0), A_partial/2(M0)  "<M0>"
  Mm_hat_partial/1(Mm_hat_partial) -> To Workspace9/1, C_hat/2(Mm_hat_partial)
  Constant/1 -> Lm_partials/2(Xi_m)
  q_m/1 -> AMA_partial/1(q_m), C_hat/1(q_m), Mm_hat_partial/1(q_m), A_partial/1(q_m), M_partials/1(q_m), Lm_partials/1(q_m)
  M_partials/3(Mm_partial) -> To Workspace6/1, Mm_hat_partial/3(Mm_partial)
  Lm_partials/2(Lm0_partial) -> To Workspace3/1, M_partials/3(Lm0_partial)
  M_partials/2(M0m_partial) -> To Workspace5/1, A_partial/4(M0m_partial)
  AMA_partial/1(AMA_partial) -> To Workspace8/1, Mm_hat_partial/2(AMA_partial)
  Bus Selector1/2 -> M_partials/5(Lm0)  "<Lm0>"
  Lm_partials/1(Lm_partial) -> To Workspace2/1, M_partials/2(Lm_partial)
  A_partial/1(A_partial) -> Out1/1, To Workspace7/1, [A_partial], AMA_partial/4(A_partial)
  C_hat/1(C_hat) -> To Workspace1/1, C_hat1/1
  M_partials/1(M0_partial) -> To Workspace4/1, AMA_partial/6(M0_partial), [M0_partial], M0_partial/1, A_partial/3(M0_partial)
  [V_I0] -> M_partials/6(V)
  Bus Selector/2 -> A_partial/5(M0m)  "<M0m>"
  q_dot_m/1 -> C_hat/3(q_dot_m)
  [V_I0] -> A_partial/6(V)
  [V_I0] -> AMA_partial/5(V)
  [A_connection] -> AMA_partial/3(A)
  [L] -> Bus Selector1/1
  Bus Selector1/1 -> M_partials/4(Lm)  "<Lm>"

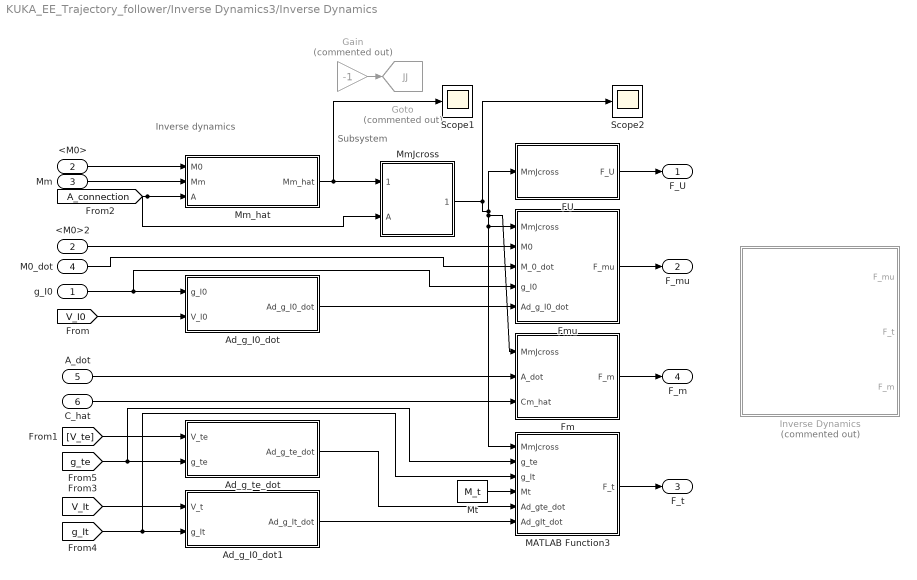
== system KUKA_EE_Trajectory_follower/Inverse Dynamics3/Inverse Dynamics ==
  note: Subsystem
  note: Inverse dynamics
  g_I0 : Inport
  <M0> : Inport  Port=2
  Mm : Inport  Port=3
  M0_dot : Inport  Port=4
  A_dot : Inport  Port=5
  C_hat : Inport  Port=6
  <M0>2 : InportShadow  Port=2
  Ad_g_I0_dot : MATLAB Function  TreatAsAtomicUnit=on
  Ad_g_I0_dot1 : MATLAB Function  TreatAsAtomicUnit=on
  Ad_g_te_dot : MATLAB Function  TreatAsAtomicUnit=on
  FU : MATLAB Function  TreatAsAtomicUnit=on
  Fm : MATLAB Function  TreatAsAtomicUnit=on
  Fmu : MATLAB Function  TreatAsAtomicUnit=on
  Gain : Gain  Commented=on  Gain=-1
  Goto : Goto  Commented=on  GotoTag=JJ  TagVisibility=global
  Inverse Dynamics : MATLAB Function  Commented=on  TreatAsAtomicUnit=on
  MATLAB Function3 : MATLAB Function  TreatAsAtomicUnit=on
  MmJcross : MATLAB Function  TreatAsAtomicUnit=on
  Mm_hat : MATLAB Function  TreatAsAtomicUnit=on
  Mt : Constant  Value=M_t
  Scope1 : Scope
  Scope2 : Scope
  F_U : Outport
  F_mu : Outport  Port=2
  F_t : Outport  Port=3
  F_m : Outport  Port=4
  wires:
  Mm/1 -> Mm_hat/2(Mm)
  [A_connection] -> Mm_hat/3(A), MmJcross/2(A)
  FU/1(F_U) -> F_U/1
  Fmu/1(F_mu) -> F_mu/1
  MATLAB Function3/1(F_t) -> F_t/1
  Fm/1(F_m) -> F_m/1
  <M0>/1 -> Mm_hat/1(M0)
  C_hat/1 -> Fm/3(Cm_hat)
  <M0>2/1 -> Fmu/2(M0)
  g_I0/1 -> Fmu/4(g_I0), Ad_g_I0_dot/1(g_I0)
  M0_dot/1 -> Fmu/3(M_0_dot)
  A_dot/1 -> Fm/2(A_dot)
  [V_I0] -> Ad_g_I0_dot/2(V_I0)
  Ad_g_I0_dot1/1(Ad_g_It_dot) -> MATLAB Function3/6(Ad_gIt_dot)
  Ad_g_I0_dot/1(Ad_g_I0_dot) -> Fmu/5(Ad_g_I0_dot)
  Ad_g_te_dot/1(Ad_g_te_dot) -> MATLAB Function3/5(Ad_gte_dot)
  [g_te] -> MATLAB Function3/2(g_te), Ad_g_te_dot/2(g_te)
  [g_It] -> MATLAB Function3/3(g_It), Ad_g_I0_dot1/2(g_It)
  [V_te] -> Ad_g_te_dot/1(V_te)
  [V_It] -> Ad_g_I0_dot1/1(V_t)
  Mt/1 -> MATLAB Function3/4(Mt)
  Mm_hat/1(Mm_hat) -> MmJcross/1(Mm_hat), Scope1/1
  MmJcross/1(MmJcross) -> FU/1(MmJcross), MATLAB Function3/1(MmJcross), Fmu/1(MmJcross), Fm/1(MmJcross), Scope2/1
  Gain/1 -> Goto/1

== system KUKA_EE_Trajectory_follower/Inverse Dynamics3/N_hat ==
  q_m : Inport
  q_dot_m : Inport  Port=2
  A : Inport  Port=3
  P : Inport  Port=4
  M0 : Inport  Port=5
  Constant : Constant  Value=iota0
  Matrix Multiply : Product  Multiplication=Matrix(*)
  N_hat : MATLAB Function  TreatAsAtomicUnit=on
  To Workspace : ToWorkspace  VariableName=N_firstpart  SaveFormat=Timeseries  SampleTime=-1
  N_hat1 : Outport
  wires:
  P/1 -> Matrix Multiply/2, N_hat/5(P)
  [M0_partial] -> N_hat/6(M0_partial)
  N_hat/1(N_hat_temp) -> To Workspace/1, Matrix Multiply/1
  q_m/1 -> N_hat/1(q_m)
  q_dot_m/1 -> N_hat/2(q_dot_m)
  [V_I0] -> N_hat/4(V)
  A/1 -> N_hat/3(A)
  [A_partial] -> N_hat/7(A_partial)
  Constant/1 -> N_hat/8(iota0)
  Matrix Multiply/1 -> N_hat1/1
  M0/1 -> N_hat/9(M0)

== system KUKA_EE_Trajectory_follower/Inverse Dynamics3/N_hat1 ==
  q_m : Inport
  q_dot_m : Inport  Port=2
  A : Inport  Port=3
  P : Inport  Port=4
  M0 : Inport  Port=5
  Constant : Constant  Value=iota0
  Matrix Multiply : Product  Multiplication=Matrix(*)
  N_hat : MATLAB Function  TreatAsAtomicUnit=on
  To Workspace : ToWorkspace  VariableName=N_firstpart  SaveFormat=Timeseries  SampleTime=-1
  N_hat1 : Outport
  wires:
  P/1 -> Matrix Multiply/2, N_hat/5(P)
  [M0_partial] -> N_hat/6(M0_partial)
  N_hat/1(N_hat_temp) -> To Workspace/1, Matrix Multiply/1
  q_m/1 -> N_hat/1(q_m)
  q_dot_m/1 -> N_hat/2(q_dot_m)
  [V_I0] -> N_hat/4(V)
  A/1 -> N_hat/3(A)
  [A_partial] -> N_hat/7(A_partial)
  Constant/1 -> N_hat/8(iota0)
  Matrix Multiply/1 -> N_hat1/1
  M0/1 -> N_hat/9(M0)

== system KUKA_EE_Trajectory_follower/PID Controller/Kinematics1 ==
  g_I0 : Inport
  g_Id : Inport  Port=2
  V_Id : Inport  Port=3
  Divide : Product  Inputs=/*  Multiplication=Matrix(*)
  Goto5 : Goto  Commented=on  GotoTag=g_Ie  TagVisibility=global
  Pose Error Function : MATLAB Function  TreatAsAtomicUnit=on
  Scope : Scope
  Scope1 : Scope
  Scope2 : Scope
  Terminator3 : Terminator
  To Workspace : ToWorkspace  VariableName=g_te  SaveFormat=Timeseries  SampleTime=-1
  Velocity_error : MATLAB Function  TreatAsAtomicUnit=on
  g_te : MATLAB Function  Commented=on  TreatAsAtomicUnit=on
  velocity of target in EE : MATLAB Function  Commented=on  TreatAsAtomicUnit=on
  g_d0 : Outport
  V_d0 : Outport  Port=2
  tag scope: g_te=global
  wires:
  g_Id/1 -> Divide/1
  g_I0/1 -> Divide/2
  Divide/1 -> g_d0/1, To Workspace/1, [g_te], Velocity_error/1(g_I0), Pose Error Function/1(g_te)
  Velocity_error/1(V_e) -> V_d0/1
  V_Id/1 -> Scope2/1, Velocity_error/3(V_It)
  [V_I0] -> Scope1/1, Velocity_error/2(V_Ie)
  Pose Error Function/1(E_g) -> Scope/1, Terminator3/1

== system KUKA_EE_Trajectory_follower/Space Manipulator1/joint//link 1 ==
  iiwa_joint_1 : sm_lib/Joints/Revolute Joint  JointMode=Normal  SenseConstraintForce=off  SenseConstraintForceX=off  SenseConstraintForceY=off  SenseConstraintForceZ=off  SenseConstraintTorque=off  SenseConstraintTorqueX=off  SenseConstraintTorqueY=off  SenseConstraintTorqueZ=off  SenseTotalForce=off  SenseTotalForceX=off  SenseTotalForceY=off  SenseTotalForceZ=off  SenseTotalTorque=off  SenseTotalTorqueX=off  SenseTotalTorqueY=off  SenseTotalTorqueZ=off  CompositeWrenchDir=FollowerOnBase  CompositeWrenchFrame=BaseFrame  EquilibriumPosition=0  EquilibriumPositionUnits=deg  SpringStiffness=0  SpringStiffnessUnits=N*m/deg  DampingCoefficient=0.5  DampingCoefficientUnits=kg*m^2/(rad*s)  TorqueActuationMode=InputTorque  MotionActuationMode=ComputedMotion  SensePosition=on  SenseVelocity=on  SenseAcceleration=on  SenseTorqueForce=off  SenseLowerLimitTorqueForce=off  SenseUpperLimitTorqueForce=off  LowerLimitSpecify=on  LowerLimitBound=-2.96705972839  LowerLimitBoundUnits=rad  LowerLimitStiffness=1e4  LowerLimitStiffnessUnits=N*m/deg  LowerLimitDamping=10  LowerLimitDampingUnits=N*m/(deg/s)  LowerLimitTransitionRegionWidth=0.1  LowerLimitTransitionRegionWidthUnits=deg  UpperLimitSpecify=on  UpperLimitBound=2.96705972839  UpperLimitBoundUnits=rad  UpperLimitStiffness=1e4  UpperLimitStiffnessUnits=N*m/deg  UpperLimitDamping=10  UpperLimitDampingUnits=N*m/(deg/s)  UpperLimitTransitionRegionWidth=0.1  UpperLimitTransitionRegionWidthUnits=deg  PositionTargetSpecify=on  PositionTargetPriority=High  PositionTargetValue=q_m(1)  PositionTargetValueUnits=rad  VelocityTargetSpecify=on  VelocityTargetPriority=High  VelocityTargetValue=q_dot_m(1)  VelocityTargetValueUnits=rad/s
  iiwa_link_1 : Subsystem
  b : PMIOPort  Side=Left
  f1 : PMIOPort  Port=2  Side=Left
  F1 : PMIOPort  Port=3  Side=Right
  q1 : PMIOPort  Port=4  Side=Right
  qd1 : PMIOPort  Port=5  Side=Right
  qdd1 : PMIOPort  Port=6  Side=Right
  connections:
  iiwa_joint_1/RConn1 -- iiwa_link_1/LConn1
  iiwa_joint_1/LConn1 -- b/RConn1
  iiwa_joint_1/RConn2 -- q1/RConn1
  f1/RConn1 -- iiwa_joint_1/LConn2
  iiwa_joint_1/RConn3 -- qd1/RConn1
  iiwa_joint_1/RConn4 -- qdd1/RConn1
  F1/RConn1 -- iiwa_link_1/RConn1

== system KUKA_EE_Trajectory_follower/Space Manipulator1/joint//link2 ==
  iiwa_joint_2 : sm_lib/Joints/Revolute Joint  JointMode=Normal  SenseConstraintForce=off  SenseConstraintForceX=off  SenseConstraintForceY=off  SenseConstraintForceZ=off  SenseConstraintTorque=off  SenseConstraintTorqueX=off  SenseConstraintTorqueY=off  SenseConstraintTorqueZ=off  SenseTotalForce=off  SenseTotalForceX=off  SenseTotalForceY=off  SenseTotalForceZ=off  SenseTotalTorque=off  SenseTotalTorqueX=off  SenseTotalTorqueY=off  SenseTotalTorqueZ=off  CompositeWrenchDir=FollowerOnBase  CompositeWrenchFrame=BaseFrame  EquilibriumPosition=0  EquilibriumPositionUnits=deg  SpringStiffness=0  SpringStiffnessUnits=N*m/deg  DampingCoefficient=0.5  DampingCoefficientUnits=kg*m^2/(rad*s)  TorqueActuationMode=InputTorque  MotionActuationMode=ComputedMotion  SensePosition=on  SenseVelocity=on  SenseAcceleration=on  SenseTorqueForce=off  SenseLowerLimitTorqueForce=off  SenseUpperLimitTorqueForce=off  LowerLimitSpecify=on  LowerLimitBound=-2.09439510239  LowerLimitBoundUnits=rad  LowerLimitStiffness=1e4  LowerLimitStiffnessUnits=N*m/deg  LowerLimitDamping=10  LowerLimitDampingUnits=N*m/(deg/s)  LowerLimitTransitionRegionWidth=0.1  LowerLimitTransitionRegionWidthUnits=deg  UpperLimitSpecify=on  UpperLimitBound=2.09439510239  UpperLimitBoundUnits=rad  UpperLimitStiffness=1e4  UpperLimitStiffnessUnits=N*m/deg  UpperLimitDamping=10  UpperLimitDampingUnits=N*m/(deg/s)  UpperLimitTransitionRegionWidth=0.1  UpperLimitTransitionRegionWidthUnits=deg  PositionTargetSpecify=on  PositionTargetPriority=High  PositionTargetValue=q_m(2)  PositionTargetValueUnits=rad  VelocityTargetSpecify=on  VelocityTargetPriority=High  VelocityTargetValue=0  VelocityTargetValueUnits=rad/s
  iiwa_link_2 : Subsystem
  b : PMIOPort  Side=Left
  F1 : PMIOPort  Port=2  Side=Right
  f2 : PMIOPort  Port=3  Side=Left
  q2 : PMIOPort  Port=4  Side=Right
  qd2 : PMIOPort  Port=5  Side=Right
  qdd2 : PMIOPort  Port=6  Side=Right
  connections:
  iiwa_joint_2/RConn3 -- qd2/RConn1
  iiwa_joint_2/RConn1 -- iiwa_link_2/LConn1
  F1/RConn1 -- iiwa_link_2/RConn1
  iiwa_joint_2/RConn4 -- qdd2/RConn1
  iiwa_joint_2/LConn1 -- b/RConn1
  f2/RConn1 -- iiwa_joint_2/LConn2
  iiwa_joint_2/RConn2 -- q2/RConn1

== system KUKA_EE_Trajectory_follower/Space Manipulator1/joint//link3 ==
  iiwa_joint_3 : sm_lib/Joints/Revolute Joint  JointMode=Normal  SenseConstraintForce=off  SenseConstraintForceX=off  SenseConstraintForceY=off  SenseConstraintForceZ=off  SenseConstraintTorque=off  SenseConstraintTorqueX=off  SenseConstraintTorqueY=off  SenseConstraintTorqueZ=off  SenseTotalForce=off  SenseTotalForceX=off  SenseTotalForceY=off  SenseTotalForceZ=off  SenseTotalTorque=off  SenseTotalTorqueX=off  SenseTotalTorqueY=off  SenseTotalTorqueZ=off  CompositeWrenchDir=FollowerOnBase  CompositeWrenchFrame=BaseFrame  EquilibriumPosition=0  EquilibriumPositionUnits=deg  SpringStiffness=0  SpringStiffnessUnits=N*m/deg  DampingCoefficient=0.5  DampingCoefficientUnits=kg*m^2/(rad*s)  TorqueActuationMode=InputTorque  MotionActuationMode=ComputedMotion  SensePosition=on  SenseVelocity=on  SenseAcceleration=on  SenseTorqueForce=off  SenseLowerLimitTorqueForce=off  SenseUpperLimitTorqueForce=off  LowerLimitSpecify=on  LowerLimitBound=-2.96705972839  LowerLimitBoundUnits=rad  LowerLimitStiffness=1e4  LowerLimitStiffnessUnits=N*m/deg  LowerLimitDamping=10  LowerLimitDampingUnits=N*m/(deg/s)  LowerLimitTransitionRegionWidth=0.1  LowerLimitTransitionRegionWidthUnits=deg  UpperLimitSpecify=on  UpperLimitBound=2.96705972839  UpperLimitBoundUnits=rad  UpperLimitStiffness=1e4  UpperLimitStiffnessUnits=N*m/deg  UpperLimitDamping=10  UpperLimitDampingUnits=N*m/(deg/s)  UpperLimitTransitionRegionWidth=0.1  UpperLimitTransitionRegionWidthUnits=deg  PositionTargetSpecify=on  PositionTargetPriority=High  PositionTargetValue=q_m(3)  PositionTargetValueUnits=rad  VelocityTargetSpecify=on  VelocityTargetPriority=High  VelocityTargetValue=0  VelocityTargetValueUnits=rad/s
  iiwa_link_3 : Subsystem
  b : PMIOPort  Side=Left
  F1 : PMIOPort  Port=2  Side=Right
  f3 : PMIOPort  Port=3  Side=Left
  q3 : PMIOPort  Port=4  Side=Right
  qd3 : PMIOPort  Port=5  Side=Right
  qdd3 : PMIOPort  Port=6  Side=Right
  connections:
  iiwa_joint_3/RConn1 -- iiwa_link_3/LConn1
  iiwa_joint_3/RConn4 -- qdd3/RConn1
  iiwa_joint_3/RConn3 -- qd3/RConn1
  iiwa_joint_3/RConn2 -- q3/RConn1
  F1/RConn1 -- iiwa_link_3/RConn1
  f3/RConn1 -- iiwa_joint_3/LConn2
  iiwa_joint_3/LConn1 -- b/RConn1

== system KUKA_EE_Trajectory_follower/Space Manipulator1/joint//link4 ==
  iiwa_joint_4 : sm_lib/Joints/Revolute Joint  JointMode=Normal  SenseConstraintForce=off  SenseConstraintForceX=off  SenseConstraintForceY=off  SenseConstraintForceZ=off  SenseConstraintTorque=off  SenseConstraintTorqueX=off  SenseConstraintTorqueY=off  SenseConstraintTorqueZ=off  SenseTotalForce=off  SenseTotalForceX=off  SenseTotalForceY=off  SenseTotalForceZ=off  SenseTotalTorque=off  SenseTotalTorqueX=off  SenseTotalTorqueY=off  SenseTotalTorqueZ=off  CompositeWrenchDir=FollowerOnBase  CompositeWrenchFrame=BaseFrame  EquilibriumPosition=0  EquilibriumPositionUnits=deg  SpringStiffness=0  SpringStiffnessUnits=N*m/deg  DampingCoefficient=0.5  DampingCoefficientUnits=kg*m^2/(rad*s)  TorqueActuationMode=InputTorque  MotionActuationMode=ComputedMotion  SensePosition=on  SenseVelocity=on  SenseAcceleration=on  SenseTorqueForce=off  SenseLowerLimitTorqueForce=off  SenseUpperLimitTorqueForce=off  LowerLimitSpecify=on  LowerLimitBound=-2.09439510239  LowerLimitBoundUnits=rad  LowerLimitStiffness=1e4  LowerLimitStiffnessUnits=N*m/deg  LowerLimitDamping=10  LowerLimitDampingUnits=N*m/(deg/s)  LowerLimitTransitionRegionWidth=0.1  LowerLimitTransitionRegionWidthUnits=deg  UpperLimitSpecify=on  UpperLimitBound=2.09439510239  UpperLimitBoundUnits=rad  UpperLimitStiffness=1e4  UpperLimitStiffnessUnits=N*m/deg  UpperLimitDamping=10  UpperLimitDampingUnits=N*m/(deg/s)  UpperLimitTransitionRegionWidth=0.1  UpperLimitTransitionRegionWidthUnits=deg  PositionTargetSpecify=on  PositionTargetPriority=High  PositionTargetValue=q_m(4)  PositionTargetValueUnits=rad  VelocityTargetSpecify=on  VelocityTargetPriority=High  VelocityTargetValue=0  VelocityTargetValueUnits=rad/s
  iiwa_link_4 : Subsystem
  b : PMIOPort  Side=Left
  F1 : PMIOPort  Port=2  Side=Right
  f4 : PMIOPort  Port=3  Side=Left
  q4 : PMIOPort  Port=4  Side=Right
  qd4 : PMIOPort  Port=5  Side=Right
  qd5 : PMIOPort  Port=6  Side=Right
  connections:
  iiwa_joint_4/RConn1 -- iiwa_link_4/LConn1
  iiwa_joint_4/RConn3 -- qd4/RConn1
  f4/RConn1 -- iiwa_joint_4/LConn2
  F1/RConn1 -- iiwa_link_4/RConn1
  iiwa_joint_4/RConn2 -- q4/RConn1
  iiwa_joint_4/LConn1 -- b/RConn1
  iiwa_joint_4/RConn4 -- qd5/RConn1

== system KUKA_EE_Trajectory_follower/Space Manipulator1/joint//link5 ==
  iiwa_joint_5 : sm_lib/Joints/Revolute Joint  JointMode=Normal  SenseConstraintForce=off  SenseConstraintForceX=off  SenseConstraintForceY=off  SenseConstraintForceZ=off  SenseConstraintTorque=off  SenseConstraintTorqueX=off  SenseConstraintTorqueY=off  SenseConstraintTorqueZ=off  SenseTotalForce=off  SenseTotalForceX=off  SenseTotalForceY=off  SenseTotalForceZ=off  SenseTotalTorque=off  SenseTotalTorqueX=off  SenseTotalTorqueY=off  SenseTotalTorqueZ=off  CompositeWrenchDir=FollowerOnBase  CompositeWrenchFrame=BaseFrame  EquilibriumPosition=0  EquilibriumPositionUnits=deg  SpringStiffness=0  SpringStiffnessUnits=N*m/deg  DampingCoefficient=0.5  DampingCoefficientUnits=kg*m^2/(rad*s)  TorqueActuationMode=InputTorque  MotionActuationMode=ComputedMotion  SensePosition=on  SenseVelocity=on  SenseAcceleration=on  SenseTorqueForce=off  SenseLowerLimitTorqueForce=off  SenseUpperLimitTorqueForce=off  LowerLimitSpecify=on  LowerLimitBound=-2.96705972839  LowerLimitBoundUnits=rad  LowerLimitStiffness=1e4  LowerLimitStiffnessUnits=N*m/deg  LowerLimitDamping=10  LowerLimitDampingUnits=N*m/(deg/s)  LowerLimitTransitionRegionWidth=0.1  LowerLimitTransitionRegionWidthUnits=deg  UpperLimitSpecify=on  UpperLimitBound=2.96705972839  UpperLimitBoundUnits=rad  UpperLimitStiffness=1e4  UpperLimitStiffnessUnits=N*m/deg  UpperLimitDamping=10  UpperLimitDampingUnits=N*m/(deg/s)  UpperLimitTransitionRegionWidth=0.1  UpperLimitTransitionRegionWidthUnits=deg  PositionTargetSpecify=on  PositionTargetPriority=High  PositionTargetValue=q_m(5)  PositionTargetValueUnits=rad  VelocityTargetSpecify=on  VelocityTargetPriority=High  VelocityTargetValue=0  VelocityTargetValueUnits=rad/s
  iiwa_link_5 : Subsystem
  b : PMIOPort  Side=Left
  F1 : PMIOPort  Port=2  Side=Right
  f5 : PMIOPort  Port=3  Side=Left
  q5 : PMIOPort  Port=4  Side=Right
  qd5 : PMIOPort  Port=5  Side=Right
  qdd5 : PMIOPort  Port=6  Side=Right
  connections:
  iiwa_joint_5/LConn1 -- b/RConn1
  iiwa_joint_5/RConn2 -- q5/RConn1
  iiwa_joint_5/RConn4 -- qdd5/RConn1
  iiwa_joint_5/RConn1 -- iiwa_link_5/LConn1
  iiwa_joint_5/RConn3 -- qd5/RConn1
  f5/RConn1 -- iiwa_joint_5/LConn2
  F1/RConn1 -- iiwa_link_5/RConn1

== system KUKA_EE_Trajectory_follower/Space Manipulator1/joint//link6 ==
  iiwa_joint_6 : sm_lib/Joints/Revolute Joint  JointMode=Normal  SenseConstraintForce=off  SenseConstraintForceX=off  SenseConstraintForceY=off  SenseConstraintForceZ=off  SenseConstraintTorque=off  SenseConstraintTorqueX=off  SenseConstraintTorqueY=off  SenseConstraintTorqueZ=off  SenseTotalForce=off  SenseTotalForceX=off  SenseTotalForceY=off  SenseTotalForceZ=off  SenseTotalTorque=off  SenseTotalTorqueX=off  SenseTotalTorqueY=off  SenseTotalTorqueZ=off  CompositeWrenchDir=FollowerOnBase  CompositeWrenchFrame=BaseFrame  EquilibriumPosition=0  EquilibriumPositionUnits=deg  SpringStiffness=0  SpringStiffnessUnits=N*m/deg  DampingCoefficient=0.5  DampingCoefficientUnits=kg*m^2/(rad*s)  TorqueActuationMode=InputTorque  MotionActuationMode=ComputedMotion  SensePosition=on  SenseVelocity=on  SenseAcceleration=on  SenseTorqueForce=off  SenseLowerLimitTorqueForce=off  SenseUpperLimitTorqueForce=off  LowerLimitSpecify=on  LowerLimitBound=-2.09439510239  LowerLimitBoundUnits=rad  LowerLimitStiffness=1e4  LowerLimitStiffnessUnits=N*m/deg  LowerLimitDamping=10  LowerLimitDampingUnits=N*m/(deg/s)  LowerLimitTransitionRegionWidth=0.1  LowerLimitTransitionRegionWidthUnits=deg  UpperLimitSpecify=on  UpperLimitBound=2.09439510239  UpperLimitBoundUnits=rad  UpperLimitStiffness=1e4  UpperLimitStiffnessUnits=N*m/deg  UpperLimitDamping=10  UpperLimitDampingUnits=N*m/(deg/s)  UpperLimitTransitionRegionWidth=0.1  UpperLimitTransitionRegionWidthUnits=deg  PositionTargetSpecify=on  PositionTargetPriority=High  PositionTargetValue=q_m(6)  PositionTargetValueUnits=rad  VelocityTargetSpecify=on  VelocityTargetPriority=High  VelocityTargetValue=0  VelocityTargetValueUnits=rad/s
  iiwa_link_6 : Subsystem
  b : PMIOPort  Side=Left
  F1 : PMIOPort  Port=2  Side=Right
  q6 : PMIOPort  Port=3  Side=Right
  f6 : PMIOPort  Port=4  Side=Left
  qd6 : PMIOPort  Port=5  Side=Right
  qdd6 : PMIOPort  Port=6  Side=Right
  connections:
  iiwa_joint_6/RConn1 -- iiwa_link_6/LConn1
  iiwa_joint_6/LConn1 -- b/RConn1
  F1/RConn1 -- iiwa_link_6/RConn1
  f6/RConn1 -- iiwa_joint_6/LConn2
  iiwa_joint_6/RConn4 -- qdd6/RConn1
  iiwa_joint_6/RConn3 -- qd6/RConn1
  iiwa_joint_6/RConn2 -- q6/RConn1
